simulink model "freedom2"  (R2015b)
settings: Solver=ode3  StartTime=0.0  StopTime=10  FixedStep=0.001  RelTol=1e-3
values from neighbouring files (symbols this model uses):
  a = 1.228    [freedom2_param.m]
  b = L-a    (= 1.172)    [freedom2_param.m]
  Iz = 2800    [freedom2_param.m]
  k1 = -51000    [freedom2_param.m]
  k2 = -40000    [freedom2_param.m]
  m = 1818.2    [freedom2_param.m]
libraries: simulink x1
settings Model: Creator=_NXP_  LastModifiedBy=_NXP_

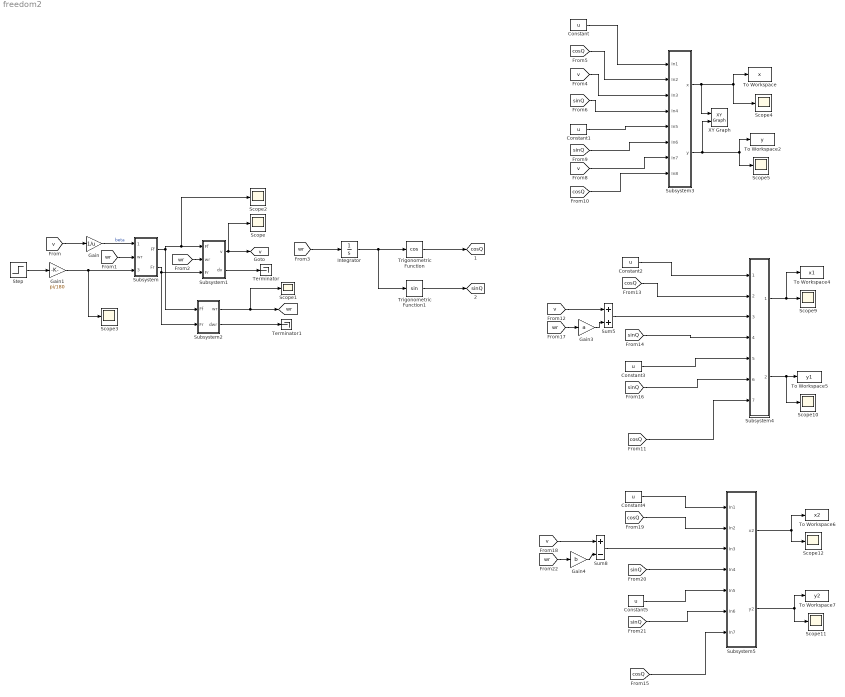
== system freedom2 ==
  Constant{,1..5} (6 alike) : Constant  Value=u
  Gain : Gain  Gain=1/u
  Gain1 : Gain  Gain=pi/180
  Gain3 : Gain  Gain=a
  Gain4 : Gain  Gain=b
  Integrator : Integrator
  Scope{,1..5,9..12} (10 alike) : Scope
  Step : Step  Time=0.05  After=8  SampleTime=0
  Subsystem : Subsystem
  Subsystem1 : Subsystem
  Subsystem2 : Subsystem
  Subsystem3 : Subsystem
  Subsystem4 : Subsystem
  Subsystem5 : Subsystem
  Sum5 : Sum
  Sum8 : Sum  Inputs=+-
  Terminator : Terminator
  Terminator1 : Terminator
  To Workspace : ToWorkspace  VariableName=x  SampleTime=-1
  To Workspace2 : ToWorkspace  VariableName=y  SampleTime=-1
  To Workspace4 : ToWorkspace  VariableName=x1  SampleTime=-1
  To Workspace5 : ToWorkspace  VariableName=y1  SampleTime=-1
  To Workspace6 : ToWorkspace  VariableName=x2  SampleTime=-1
  To Workspace7 : ToWorkspace  VariableName=y2  SampleTime=-1
  Trigonometric Function : Trigonometry  Operator=cos
  Trigonometric Function1 : Trigonometry
  XY Graph : simulink/Sinks/XY Graph  xmin=-10  xmax=30  ymin=-5  ymax=35  st=-1
  tag scope: cosQ=global, sinQ=global, v=global, wr=global
  wires:
  Gain/1 -> Subsystem/1(beat)  "beta"
  Gain1/1 -> Scope3/1, Subsystem/3(deta)
  Subsystem/1(Ff) -> Subsystem2/1(Ff), Scope2/1, Subsystem1/1(Ff)
  Subsystem/2(Fr) -> Subsystem2/2(Fr), Subsystem1/3(Fr)
  Subsystem1/1(v) -> Scope/1, [v]
  Subsystem2/1(wr) -> Scope1/1, [wr]
  Step/1 -> Gain1/1
  Subsystem1/2(dv) -> Terminator/1
  Subsystem2/2(dwr) -> Terminator1/1
  [v] -> Gain/1
  [wr] -> Subsystem/2(wr)
  [wr] -> Subsystem1/2(wr)
  [wr] -> Integrator/1
  Integrator/1 -> Trigonometric Function1/1, Trigonometric Function/1
  Trigonometric Function/1 -> [cosQ]
  Trigonometric Function1/1 -> [sinQ]
  [v] -> Sum5/1
  [wr] -> Gain3/1
  Gain3/1 -> Sum5/2
  [v] -> Sum8/1
  [wr] -> Gain4/1
  Gain4/1 -> Sum8/2
  Subsystem3/2(y) -> XY Graph/2, Scope5/1, To Workspace2/1
  Subsystem3/1(x) -> XY Graph/1, Scope4/1, To Workspace/1
  Constant/1 -> Subsystem3/1(In1)
  [cosQ] -> Subsystem3/2(In2)
  [v] -> Subsystem3/3(In3)
  [sinQ] -> Subsystem3/4(In4)
  Constant1/1 -> Subsystem3/5(In5)
  [sinQ] -> Subsystem3/6(In6)
  [v] -> Subsystem3/7(In7)
  [cosQ] -> Subsystem3/8(In8)
  Subsystem4/1(x1) -> To Workspace4/1, Scope9/1
  Subsystem4/2(y1) -> Scope10/1, To Workspace5/1
  Constant2/1 -> Subsystem4/1(In1)
  [cosQ] -> Subsystem4/2(In2)
  Sum5/1 -> Subsystem4/3(In3)
  [sinQ] -> Subsystem4/4(In4)
  Constant3/1 -> Subsystem4/5(In5)
  [sinQ] -> Subsystem4/6(In6)
  [cosQ] -> Subsystem4/7(In7)
  Subsystem5/1(x2) -> Scope12/1, To Workspace6/1
  Subsystem5/2(y2) -> To Workspace7/1, Scope11/1
  Constant4/1 -> Subsystem5/1(In1)
  [cosQ] -> Subsystem5/2(In2)
  Sum8/1 -> Subsystem5/3(In3)
  [sinQ] -> Subsystem5/4(In4)
  Constant5/1 -> Subsystem5/5(In5)
  [sinQ] -> Subsystem5/6(In6)
  [cosQ] -> Subsystem5/7(In7)

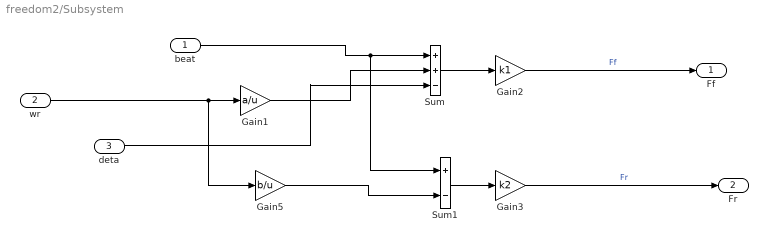
== system freedom2/Subsystem ==
  beat : Inport
  wr : Inport  Port=2
  deta : Inport  Port=3
  Gain1 : Gain  Gain=a/u
  Gain2 : Gain  Gain=k1
  Gain3 : Gain  Gain=k2
  Gain5 : Gain  Gain=b/u
  Sum : Sum  Inputs=++-
  Sum1 : Sum  Inputs=+-
  Ff : Outport
  Fr : Outport  Port=2
  wires:
  Gain5/1 -> Sum1/2
  beat/1 -> Sum1/1, Sum/1
  Sum/1 -> Gain2/1
  wr/1 -> Gain5/1, Gain1/1
  Gain1/1 -> Sum/2
  Gain2/1 -> Ff/1  "Ff"
  deta/1 -> Sum/3
  Sum1/1 -> Gain3/1
  Gain3/1 -> Fr/1  "Fr"

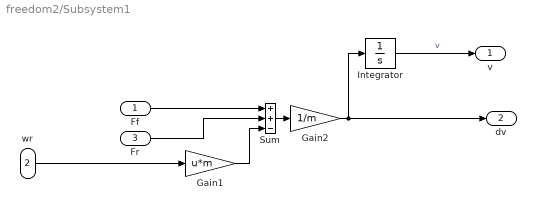
== system freedom2/Subsystem1 ==
  Ff : Inport
  wr : Inport  Port=2
  Fr : Inport  Port=3
  Gain1 : Gain  Gain=u*m
  Gain2 : Gain  Gain=1/m
  Integrator : Integrator
  Sum : Sum  Inputs=++-
  v : Outport
  dv : Outport  Port=2
  wires:
  Gain2/1 -> dv/1, Integrator/1
  Fr/1 -> Sum/2
  Ff/1 -> Sum/1
  Gain1/1 -> Sum/3
  Sum/1 -> Gain2/1
  Integrator/1 -> v/1  "v"
  wr/1 -> Gain1/1

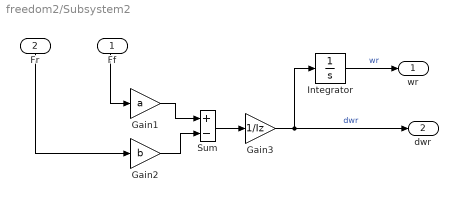
== system freedom2/Subsystem2 ==
  Ff : Inport
  Fr : Inport  Port=2
  Gain1 : Gain  Gain=a
  Gain2 : Gain  Gain=b
  Gain3 : Gain  Gain=1/Iz
  Integrator : Integrator
  Sum : Sum  Inputs=+-
  wr : Outport
  dwr : Outport  Port=2
  wires:
  Sum/1 -> Gain3/1
  Gain3/1 -> dwr/1, Integrator/1  "dwr"
  Integrator/1 -> wr/1  "wr"
  Gain2/1 -> Sum/2
  Fr/1 -> Gain2/1
  Ff/1 -> Gain1/1
  Gain1/1 -> Sum/1

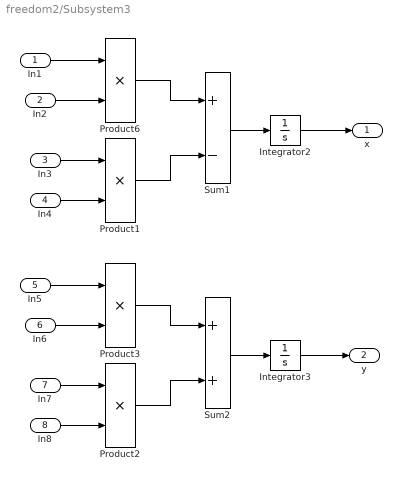
== system freedom2/Subsystem3 ==
  In1 : Inport
  In2 : Inport  Port=2
  In3 : Inport  Port=3
  In4 : Inport  Port=4
  In5 : Inport  Port=5
  In6 : Inport  Port=6
  In7 : Inport  Port=7
  In8 : Inport  Port=8
  Integrator2 : Integrator
  Integrator3 : Integrator
  Product{1..3,6} (4 alike) : Product  Inputs=**  RndMeth=Zero
  Sum1 : Sum  Inputs=+-
  Sum2 : Sum
  x : Outport
  y : Outport  Port=2
  wires:
  Sum1/1 -> Integrator2/1
  Product6/1 -> Sum1/1
  In1/1 -> Product6/1
  In2/1 -> Product6/2
  In3/1 -> Product1/1
  Product1/1 -> Sum1/2
  In4/1 -> Product1/2
  Integrator2/1 -> x/1
  In8/1 -> Product2/2
  Product3/1 -> Sum2/1
  In5/1 -> Product3/1
  Sum2/1 -> Integrator3/1
  In6/1 -> Product3/2
  In7/1 -> Product2/1
  Integrator3/1 -> y/1
  Product2/1 -> Sum2/2

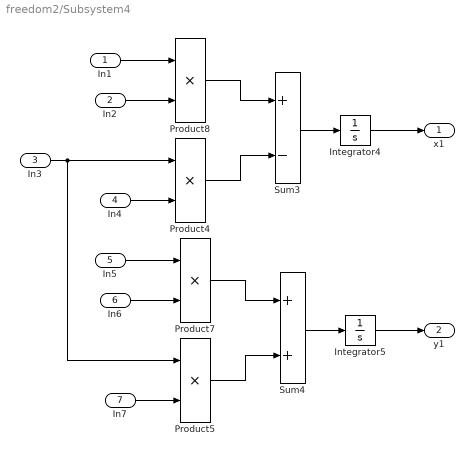
== system freedom2/Subsystem4 ==
  In1 : Inport
  In2 : Inport  Port=2
  In3 : Inport  Port=3
  In4 : Inport  Port=4
  In5 : Inport  Port=5
  In6 : Inport  Port=6
  In7 : Inport  Port=7
  Integrator4 : Integrator
  Integrator5 : Integrator
  Product{4..5,7..8} (4 alike) : Product  Inputs=**  RndMeth=Zero
  Sum3 : Sum  Inputs=+-
  Sum4 : Sum
  x1 : Outport
  y1 : Outport  Port=2
  wires:
  In1/1 -> Product8/1
  Sum3/1 -> Integrator4/1
  Integrator5/1 -> y1/1
  In7/1 -> Product5/2
  Sum4/1 -> Integrator5/1
  In6/1 -> Product7/2
  Product7/1 -> Sum4/1
  Product5/1 -> Sum4/2
  In2/1 -> Product8/2
  In4/1 -> Product4/2
  Product8/1 -> Sum3/1
  Product4/1 -> Sum3/2
  In5/1 -> Product7/1
  Integrator4/1 -> x1/1
  In3/1 -> Product5/1, Product4/1

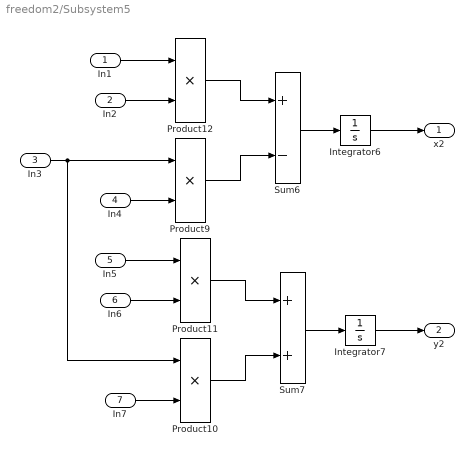
== system freedom2/Subsystem5 ==
  In1 : Inport
  In2 : Inport  Port=2
  In3 : Inport  Port=3
  In4 : Inport  Port=4
  In5 : Inport  Port=5
  In6 : Inport  Port=6
  In7 : Inport  Port=7
  Integrator6 : Integrator
  Integrator7 : Integrator
  Product{9..12} (4 alike) : Product  Inputs=**  RndMeth=Zero
  Sum6 : Sum  Inputs=+-
  Sum7 : Sum
  x2 : Outport
  y2 : Outport  Port=2
  wires:
  In7/1 -> Product10/2
  In2/1 -> Product12/2
  Sum7/1 -> Integrator7/1
  Product11/1 -> Sum7/1
  Integrator7/1 -> y2/1
  In1/1 -> Product12/1
  Product12/1 -> Sum6/1
  In5/1 -> Product11/1
  Product10/1 -> Sum7/2
  In6/1 -> Product11/2
  Product9/1 -> Sum6/2
  Sum6/1 -> Integrator6/1
  Integrator6/1 -> x2/1
  In3/1 -> Product10/1, Product9/1
  In4/1 -> Product9/2
